simulink model "PLCPneumaticCylinder"  (R2017b)
settings: Solver=VariableStepAuto  StartTime=0.0  StopTime=inf  RelTol=1e-3
libraries: library_plc2simulink x15
settings Model: Creator=Moritz  LastModifiedBy=Moritz
settings DataIOCC: ReturnWorkspaceOutputs=on
settings SFSimCC: SimUseLocalCustomCode=on
settings RTWCC: RTWUseLocalCustomCode=on

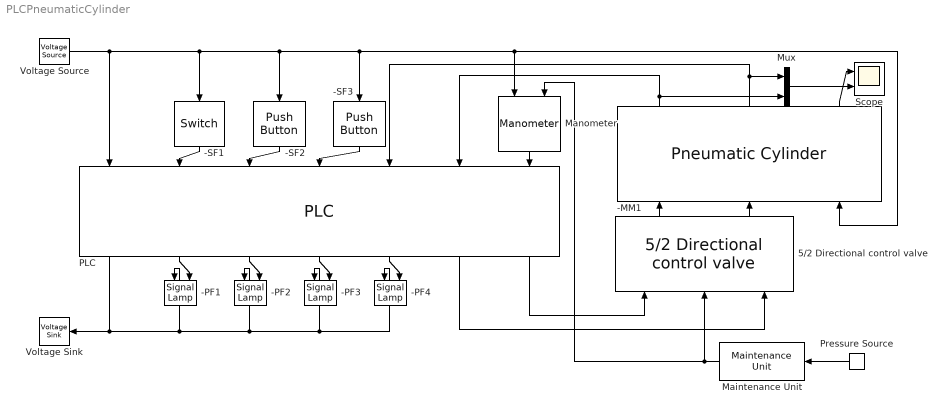
== system PLCPneumaticCylinder ==
  -MM1 : library_plc2simulink/Pneumatic Cylinder  minPos=0  maxPos=100  pistonSpeed=200  currentPos=-1.0914e-10  updateIcon=0.1
      settings: SourceProductName=PLC2Simulink
  -PF1 : library_plc2simulink/Signal Lamp  Value=off  updateTime=0.1  colorOn=[0.2,1,0.2]  colorOff=[1,1,1]
      settings: SourceProductName=PLC2Simulink
  -PF2 : library_plc2simulink/Signal Lamp  Value=off  updateTime=0.1  colorOn=[1,1,0.2]  colorOff=[1,1,1]
      settings: SourceProductName=PLC2Simulink
  -PF3 : library_plc2simulink/Signal Lamp  Value=on  updateTime=0.1  colorOn=[1,1,0.2]  colorOff=[1,1,1]
      settings: SourceProductName=PLC2Simulink
  -PF4 : library_plc2simulink/Signal Lamp  Value=off  updateTime=0.1  colorOn=[1,0.2,0.2]  colorOff=[1,1,1]
      settings: SourceProductName=PLC2Simulink
  -SF1 : library_plc2simulink/Switch  Gain=1  Multiplication=Element-wise(K.*u)  ParamMin=[]  ParamMax=[]  OutMin=[]  OutMax=[]  SampleTime=-1
      settings: SourceProductName=PLC2Simulink
  -SF2 : library_plc2simulink/Push Button  deactTime=0.3  StateOn=0
      settings: SourceProductName=PLC2Simulink
  -SF3 : library_plc2simulink/Push Button  deactTime=0.3  StateOn=0
      settings: SourceProductName=PLC2Simulink
  5/2 Directional control valve : library_plc2simulink/5//2 Directional control valve  updateIcon=0.1  state=0
      settings: SourceProductName=PLC2Simulink
  Maintenance Unit : library_plc2simulink/Maintenance Unit  pressure=0.300
      settings: SourceProductName=PLC2Simulink
  "Manometer " : library_plc2simulink/Manometer   stateOn=0  updateIcon=0.1  actPressure=0.500
      settings: SourceProductName=PLC2Simulink
  Mux : Mux  Inputs=2
  PLC : library_plc2simulink/PLC  instanceName=PLC1  numInputs=6  numOutputs=6  timeStep=0.05  externalSupplyVoltage=on
      settings: SourceProductName=PLC2Simulink
  Pressure Source : library_plc2simulink/Pressure Source  pressure=5
      settings: SourceProductName=PLC2Simulink
  Scope : Scope  NumInputPorts=2
  Voltage Sink : library_plc2simulink/Voltage Sink
      settings: SourceProductName=PLC2Simulink
  Voltage Source : library_plc2simulink/Voltage Source  voltage=24
      settings: SourceProductName=PLC2Simulink
  wires:
  -MM1/3 -> Scope/1
  Pressure Source/1 -> Maintenance Unit/1
  Maintenance Unit/1 -> "Manometer "/1, 5/2 Directional control valve/2
  5/2 Directional control valve/1 -> -MM1/1
  5/2 Directional control valve/2 -> -MM1/2
  -SF3/1 -> PLC/4
  Voltage Source/1 -> -MM1/3, "Manometer "/2, -SF3/1, -SF2/1, -SF1/1, PLC/1
  PLC/3 -> -PF2/1
  -SF1/1 -> PLC/2
  -SF2/1 -> PLC/3
  -MM1/1 -> PLC/6, Mux/2
  -MM1/2 -> PLC/5, Mux/1
  PLC/1 -> -PF4/2, -PF3/2, -PF2/2, -PF1/2, Voltage Sink/1
  PLC/2 -> -PF1/1
  PLC/7 -> 5/2 Directional control valve/1
  PLC/6 -> 5/2 Directional control valve/3
  PLC/4 -> -PF3/1
  Mux/1 -> Scope/2
  "Manometer "/1 -> PLC/7
  PLC/5 -> -PF4/1
